simulink model "vtol50kg_airframe"  (R2024b)
settings: Solver=FixedStepAuto  StartTime=0  StopTime=200  FixedStep=5/1000  RelTol=1e-3
model workspace (MAT data in the model file):
  Sig = Simulink.Signal
  Sig.Dimensions = -1
  Sig.DimensionsMode = 'auto'
  Sig.Complexity = 'auto'
  Sig.SampleTime = -1
  Sig.SamplingMode = 'auto'
  Sig.DataType = 'auto'
  Sig1 = Simulink.Signal
  Sig1.Dimensions = -1
  Sig1.DimensionsMode = 'auto'
  Sig1.Complexity = 'auto'
  Sig1.SampleTime = -1
  Sig1.SamplingMode = 'auto'
  Sig1.DataType = 'auto'
  Sig2 = Simulink.Signal
  Sig2.Dimensions = -1
  Sig2.DimensionsMode = 'auto'
  Sig2.Complexity = 'auto'
  Sig2.SampleTime = -1
  Sig2.SamplingMode = 'auto'
  Sig2.DataType = 'auto'
  Sig3 = Simulink.Signal
  Sig3.Dimensions = -1
  Sig3.DimensionsMode = 'auto'
  Sig3.Complexity = 'auto'
  Sig3.SampleTime = -1
  Sig3.SamplingMode = 'auto'
  Sig3.DataType = 'auto'
  Sig4 = Simulink.Signal
  Sig4.Dimensions = -1
  Sig4.DimensionsMode = 'auto'
  Sig4.Complexity = 'auto'
  Sig4.SampleTime = -1
  Sig4.SamplingMode = 'auto'
  Sig4.DataType = 'auto'
  Sig5 = Simulink.Signal
  Sig5.Dimensions = -1
  Sig5.DimensionsMode = 'auto'
  Sig5.Complexity = 'auto'
  Sig5.SampleTime = -1
  Sig5.SamplingMode = 'auto'
  Sig5.DataType = 'auto'
  Sig6 = Simulink.Signal
  Sig6.Dimensions = -1
  Sig6.DimensionsMode = 'auto'
  Sig6.Complexity = 'auto'
  Sig6.SampleTime = -1
  Sig6.SamplingMode = 'auto'
  Sig6.DataType = 'auto'
values from neighbouring files (symbols this model uses):
  aerody =     [vtol50kg_airframe_data.mat]    (also in vtol50kg_airframe_init.m = init_aerody; vtol50kg_initdata.m = init_aerody)
  engine =     [vtol50kg_airframe_data.mat]    (also in vtol50kg_airframe_init.m = init_engine; vtol50kg_initdata.m = init_engine)
  mass =     [vtol50kg_airframe_data.mat]    (also in vtol50kg_airframe_init.m = init_weight; vtol50kg_initdata.m = init_weight)
  motor =     [vtol50kg_airframe_data.mat]    (also in vtol50kg_airframe_init.m = init_motor; vtol50kg_initdata.m = init_motor)
  payload =     [vtol50kg_airframe_data.mat]    (also in vtol50kg_airframe_init.m = init_payload; vtol50kg_initdata.m = init_payload)
undefined symbols (not defined in the file or in its folder): convertTo, datetime, Earth, F, Light, MIL, plant, WGS84, WMM2020
libraries: aerolibconvert2 x5, aerolibasang x5, aerolibwind2 x3, aerolibactuator x2, shared6dof x1, matrix_library x1, aerolibatmos2 x1, aerolibtransform2 x1, aerolibgravity2 x1
(part 1 of 2)
settings Model: DataDictionary=nextpilot_datadict.sldd  PauseTimes=10  Creator=zhanfuyu  LastModifiedBy=CETCA
settings OptimizationCC: BlockReduction=off  OptimizeBlockIOStorage=off  BufferReuse=off  ReuseModelBlockBuffer=off
settings DebuggingCC: AlgebraicLoopMsg=none
settings RTWCC: GPUComputeCapability=3.5

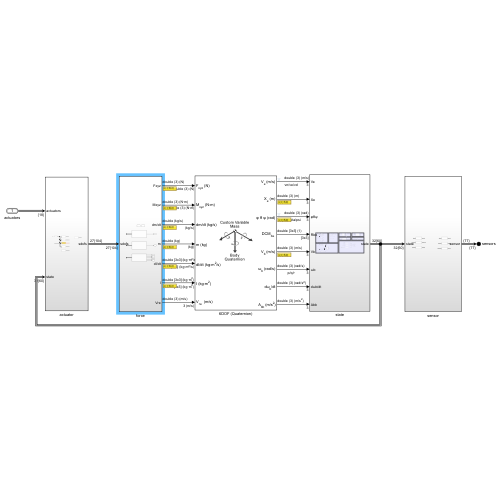
[thumbnail: Simulink's stored preview of the top-level diagram]
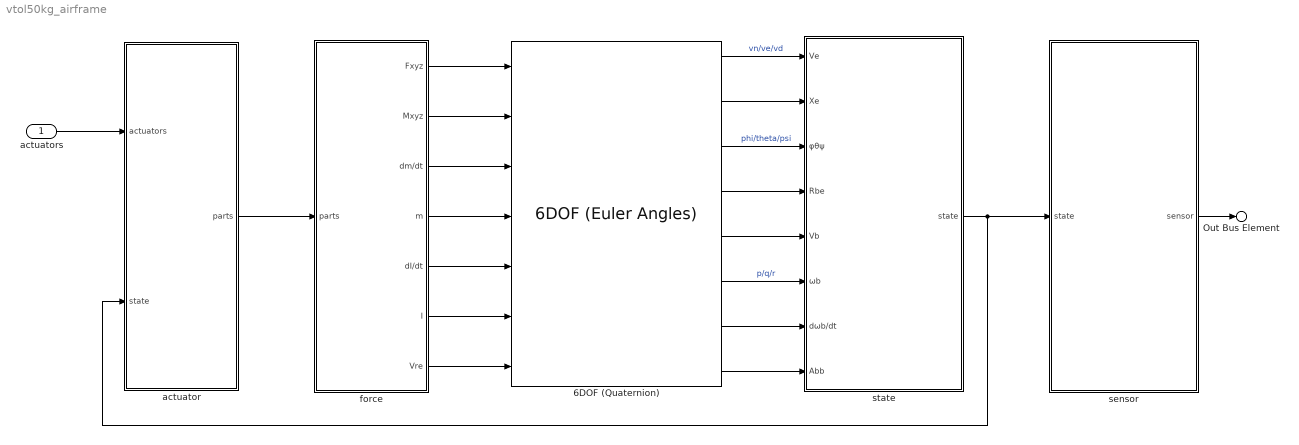
== system vtol50kg_airframe ==
  actuators : Inport  OutDataTypeStr=Bus: actuator_outputs_s
  6DOF (Quaternion) : shared6dof/6DOF (Euler Angles)  units=Metric (MKS)  mtype=Custom Variable  rep=Quaternion  xme_0=[0 0 0]  Vm_0=plant.init.vx_vy_vz  eul_0=plant.init.phi_theta_psi  pm_0=plant.init.p_q_r  mass_0=47  mass_e=0.5  mass_f=2.0  inertia=mass.emtpy_inertia  inertia_e=eye(3)  inertia_f=2*eye(3)  k_quat=1.0  vre_flag=on  abi_flag=off  aMode=0  xme_statename=''  Vm_statename=''  eul_statename=''  quat_statename=''  pm_statename=''  mass_statename=''
      settings: LibrarySourceBlock=aerolib6dof2/6DOF (Quaternion)
  actuator : Subsystem
  force : Subsystem
  sensor : Subsystem
  state : Subsystem
  Out Bus Element : Outport  PortName=sensors
  wires:
  state/1(state) -> actuator/2(state), sensor/1(state)
  sensor/1(sensor) -> Out Bus Element/1
  actuators/1 -> actuator/1(actuators)
  actuator/1(parts) -> force/1(parts)
  6DOF (Quaternion)/1 -> state/1(Ve)  "vn/ve/vd"
  6DOF (Quaternion)/2 -> state/2(Xe)
  6DOF (Quaternion)/3 -> state/3(φθψ)  "phi/theta/psi"
  6DOF (Quaternion)/4 -> state/4(Rbe)
  6DOF (Quaternion)/5 -> state/5(Vb)
  6DOF (Quaternion)/6 -> state/6(ωb)  "p/q/r"
  6DOF (Quaternion)/7 -> state/7(dωb/dt)
  6DOF (Quaternion)/8 -> state/8(Abb)
  force/1(Fxyz) -> 6DOF (Quaternion)/1
  force/2(Mxyz) -> 6DOF (Quaternion)/2
  force/3(dm/dt) -> 6DOF (Quaternion)/3
  force/4(m) -> 6DOF (Quaternion)/4
  force/5(dI/dt) -> 6DOF (Quaternion)/5
  force/6(I) -> 6DOF (Quaternion)/6
  force/7(Vre) -> 6DOF (Quaternion)/7

== system vtol50kg_airframe/actuator ==
  Bus Element In1 : Inport  PortName=actuators  Element=output
  Bus Element In : Inport  Port=2  PortName=state
  Subsystem : Subsystem
  battery : Subsystem
  engine : Subsystem
  fixed wing : Subsystem
  landgear : Subsystem
  payload : Subsystem
  rotor copter : Subsystem
  Bus Element Out : Outport  PortName=parts  Element=aerody
  Bus Element Out1 : Outport  PortName=parts  Element=rotor
  Bus Element Out2 : Outport  PortName=parts  Element=engine
  Bus Element Out3 : Outport  PortName=parts  Element=landgear
  Bus Element Out4 : Outport  PortName=parts  Element=battery
  Bus Element Out5 : Outport  PortName=parts  Element=payload
  wires:
  Bus Element In1/1 -> Subsystem/1(actuator)
  Subsystem/1(command) -> landgear/1(cmd), engine/1(cmd), rotor copter/1(cmd), fixed wing/1(cmd)
  Bus Element In/1 -> landgear/2(state), fixed wing/2(state), rotor copter/2(state), engine/2(state)
  fixed wing/1(aerody) -> Bus Element Out/1
  rotor copter/1(rotor) -> Bus Element Out1/1
  engine/1(engine) -> Bus Element Out2/1
  landgear/1(landgear) -> Bus Element Out3/1
  battery/1(battery) -> Bus Element Out4/1
  payload/1(payload) -> Bus Element Out5/1

== system vtol50kg_airframe/force ==
  BusElementIn : Inport  PortName=parts
  BusElementIn1 : Inport  PortName=parts
  BusElementIn2 : Inport  PortName=parts
  Force : Subsystem
  Goto Tag Visibility : GotoTagVisibility  GotoTag=mass
  Goto Tag Visibility1 : GotoTagVisibility  GotoTag=cog
  "Mass " : Subsystem
  Moment : Subsystem
  Fxyz : Outport
  Mxyz : Outport  Port=2
  dm/dt : Outport  Port=3
  m : Outport  Port=4
  dI/dt : Outport  Port=5
  I : Outport  Port=6
  Vre : Outport  Port=7
  wires:
  Force/1(Fxyz) -> Fxyz/1  "Fxzy"
  Moment/1(Mxyz) -> Mxyz/1  "Mxyz"
  BusElementIn/1 -> Force/1(parts)
  BusElementIn1/1 -> Moment/1(parts)
  BusElementIn2/1 -> "Mass "/1(parts)
  "Mass "/1(dM/dt) -> dm/dt/1
  "Mass "/2(M) -> m/1
  "Mass "/3(dI/dt) -> dI/dt/1
  "Mass "/4(I) -> I/1
  "Mass "/5(Vre) -> Vre/1

== system vtol50kg_airframe/sensor ==
  Bus Element In{,1..5} (6 alike) : Inport  PortName=state
  accel : Subsystem
  airspeed : Subsystem
  baro : Subsystem
  gps : Subsystem
  gyro : Subsystem
  mag : Subsystem
  Bus Element Out1 : Outport  PortName=sensor  Element=gps
  Bus Element Out3 : Outport  PortName=sensor  Element=gyro
  Bus Element Out4 : Outport  PortName=sensor  Element=accel
  Bus Element Out : Outport  PortName=sensor  Element=mag
  Bus Element Out2 : Outport  PortName=sensor  Element=baro
  Bus Element Out5 : Outport  PortName=sensor  Element=dpressure
  wires:
  Bus Element In/1 -> gps/1(state)
  Bus Element In1/1 -> mag/1(state)
  mag/1(mag) -> Bus Element Out/1
  gps/1(gps) -> Bus Element Out1/1
  baro/1(baro) -> Bus Element Out2/1
  Bus Element In2/1 -> baro/1(state)
  Bus Element In3/1 -> gyro/1(state)
  gyro/1(gyro) -> Bus Element Out3/1
  Bus Element In4/1 -> accel/1(state)
  accel/1(accel) -> Bus Element Out4/1
  Bus Element In5/1 -> airspeed/1(state)
  airspeed/1(dpressure) -> Bus Element Out5/1

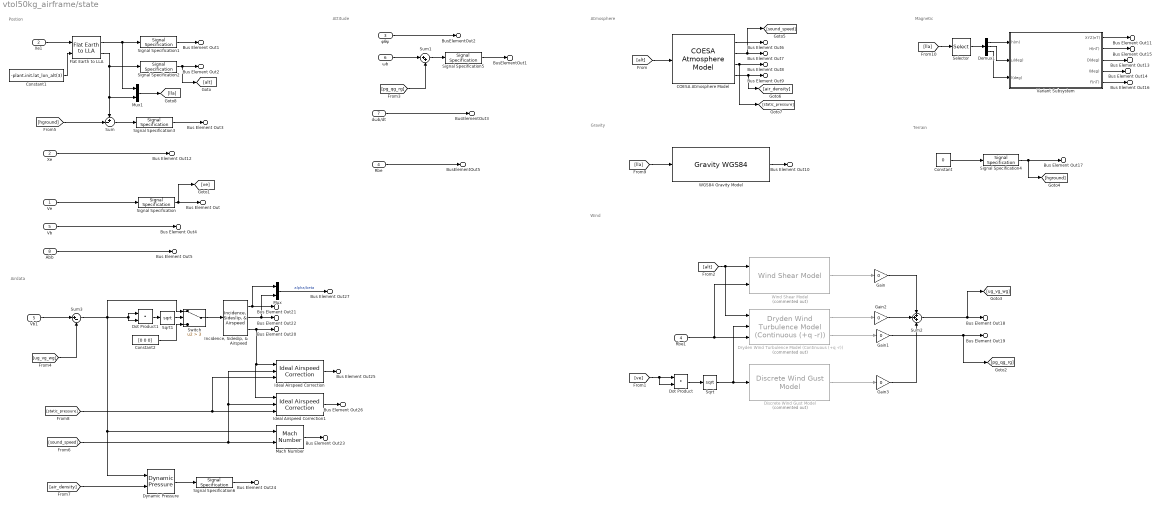
== system vtol50kg_airframe/state ==
  note: Postion
  note: Attitude
  note: Atmosphere
  note: Gravity
  note: Magnetic
  note: Terrain
  note: Wind
  note: Airdata
  Ve : Inport
  Xe : Inport  Port=2
  φθψ : Inport  Port=3
  Rbe : Inport  Port=4
  Vb : Inport  Port=5
  ωb : Inport  Port=6
  dωb/dt : Inport  Port=7
  Abb : Inport  Port=8
  COESA Atmosphere Model : aerolibatmos2/COESA Atmosphere Model  units=Metric (MKS)  spec=1976 COESA-extended U.S. Standard Atmosphere  model=Profile  profile_var=High temperature  profile_percent=1%  profile_alt=5 km (16404 ft)  envelope_var=High temperature  envelope_percent=1%  action=Warning
  Constant : Constant  Value=0
  Constant1 : Constant  Value=-plant.init.lat_lon_alt(3)
  Constant2 : Constant  Value=[0 0 0]
  Demux1 : Demux  Outputs=3
  Discrete Wind Gust Model : aerolibwind2/Discrete Wind Gust Model  Commented=on  units=Metric (MKS)  Gx=on  Gy=on  Gz=on  t_0=5  d_m=[120 120 80]  v_m=[3.5 3.5 3.0]
  Dot Product : DotProduct  OutDataTypeStr=Inherit: Inherit via internal rule
  Dot Product1 : DotProduct  OutDataTypeStr=Inherit: Inherit via internal rule
  Dryden Wind Turbulence Model (Continuous (+q -r)) : aerolibwind2/Dryden Wind Turbulence Model  (Continuous (+q -r))  Commented=on  units=Metric (MKS)  spec=MIL-F-8785C  model=Continuous Dryden (+q -r)  W20=15  Wdeg=0  TurbProb=10^-2 - Light  L_high=533.4  Wingspan=10  ts=0.1  Seed=[23341 23342 23343 23344]  T_on=on
  Dynamic Pressure : aerolibasang/Dynamic Pressure
  Flat Earth to LLA : aerolibtransform2/Flat Earth to LLA  units=Metric (MKS)  ptype=Earth (WGS84)  F=1/298.257223563  R=6378137  refPosPort=off  LL0=plant.init.lat_lon_alt(1:2)  psi=0
  Gain{,1..3} (4 alike) : Gain  Gain=0
  Ideal Airspeed Correction : aerolibasang/Ideal Airspeed Correction  units=Metric (MKS)  vel_in=TAS  vel_out_tas=CAS  vel_out_eas=TAS  vel_out_cas=TAS  method=Table Lookup  SubOnly=off  action=None
  Ideal Airspeed Correction1 : aerolibasang/Ideal Airspeed Correction  units=Metric (MKS)  vel_in=TAS  vel_out_tas=EAS  vel_out_eas=TAS  vel_out_cas=TAS  method=Table Lookup  SubOnly=off  action=None
  "Incidence, Sideslip, & Airspeed" : aerolibasang/Incidence, Sideslip, & Airspeed
  Mach Number : aerolibasang/Mach Number
  Mux : Mux  Inputs=2
  Mux1 : Mux  Inputs=2
  Rbe1 : InportShadow  Port=4
  Selector : Selector  InputPortWidth=3  IndexOptions=Index vector (dialog)  Indices=[3 1 2]  OutputSizes=1
  Signal Specification : SignalSpecification  Unit=m/s
  Signal Specification1 : SignalSpecification  Unit=deg
  Signal Specification2 : SignalSpecification  Unit=m
  Signal Specification3 : SignalSpecification  Unit=m
  Signal Specification4 : SignalSpecification  Unit=m
  Signal Specification5 : SignalSpecification  Unit=rad/s
  Signal Specification6 : SignalSpecification  Unit=Pa
  Sqrt : Sqrt
  Sqrt1 : Sqrt
  Sum : Sum  Inputs=+-|
  Sum1 : Sum  Inputs=|++
  Sum2 : Sum  Inputs=+++
  Sum3 : Sum  Inputs=|+-
  Switch : Switch  Criteria=u2 > Threshold  Threshold=3  SaturateOnIntegerOverflow=off  InputSameDT=off
  Variant Subsystem : Subsystem  Variant=on
  Vb1 : InportShadow  Port=5
  "WGS84 Gravity Model  " : GravityWGS84
  Wind Shear Model : aerolibwind2/Wind Shear Model  Commented=on  units=Metric (MKS)  phase=Category C - Terminal Flight Phase  W_20=15  Wdeg=0
  Xe1 : InportShadow  Port=2
  Bus Element Out1 : Outport  PortName=state  Element=aircraft.position.lat_lon
  Bus Element Out2 : Outport  PortName=state  Element=aircraft.position.alt
  Bus Element Out3 : Outport  PortName=state  Element=aircraft.position.agl
  Bus Element Out12 : Outport  PortName=state  Element=aircraft.position.pn_pe_pd
  Bus Element Out : Outport  PortName=state  Element=aircraft.position.vn_ve_vd
  Bus Element Out4 : Outport  PortName=state  Element=aircraft.position.ub_vb_wb
  Bus Element Out5 : Outport  PortName=state  Element=aircraft.position.ax_ay_az
  BusElementOut2 : Outport  PortName=state  Element=aircraft.attitude.phi_theta_psi
  BusElementOut1 : Outport  PortName=state  Element=aircraft.attitude.p_q_r
  BusElementOut3 : Outport  PortName=state  Element=aircraft.attitude.pdot_qdot_rdot
  BusElementOut5 : Outport  PortName=state  Element=aircraft.attitude.Rbe
  Bus Element Out20 : Outport  PortName=state  Element=aircraft.airdata.airspeed
  Bus Element Out21 : Outport  PortName=state  Element=aircraft.airdata.alpha
  Bus Element Out22 : Outport  PortName=state  Element=aircraft.airdata.beta
  Bus Element Out23 : Outport  PortName=state  Element=aircraft.airdata.mach
  Bus Element Out24 : Outport  PortName=state  Element=aircraft.airdata.qbar
  Bus Element Out25 : Outport  PortName=state  Element=aircraft.airdata.airspeed_cali
  Bus Element Out26 : Outport  PortName=state  Element=aircraft.airdata.airspeed_equ
  Bus Element Out27 : Outport  PortName=state  Element=aircraft.airdata.alpha_beta
  Bus Element Out6 : Outport  PortName=state  Element=environ.atmosphere.temperature
  Bus Element Out7 : Outport  PortName=state  Element=environ.atmosphere.soundspeed
  Bus Element Out8 : Outport  PortName=state  Element=environ.atmosphere.pressure
  Bus Element Out9 : Outport  PortName=state  Element=environ.atmosphere.density
  Bus Element Out10 : Outport  PortName=state  Element=environ.gravity.xyz
  Bus Element Out11 : Outport  PortName=state  Element=environ.magnetic.xyz
  Bus Element Out13 : Outport  PortName=state  Element=environ.magnetic.declination
  Bus Element Out14 : Outport  PortName=state  Element=environ.magnetic.inclination
  Bus Element Out15 : Outport  PortName=state  Element=environ.magnetic.hor_intensity
  Bus Element Out16 : Outport  PortName=state  Element=environ.magnetic.total_intensity
  Bus Element Out17 : Outport  PortName=state  Element=environ.terrain.hground
  Bus Element Out18 : Outport  PortName=state  Element=environ.wind.ug_vg_wg
  Bus Element Out19 : Outport  PortName=state  Element=environ.wind.pg_qg_rg
  wires:
  Signal Specification6/1 -> Bus Element Out24/1
  Signal Specification5/1 -> BusElementOut1/1
  Gain3/1 -> Sum2/3
  Gain2/1 -> Sum2/2
  Gain/1 -> Sum2/1
  Mux/1 -> Bus Element Out27/1  "alpha/beta"
  Ideal Airspeed Correction1/1 -> Bus Element Out26/1
  Ideal Airspeed Correction/1 -> Bus Element Out25/1
  [static_pressure] -> Ideal Airspeed Correction1/3, Ideal Airspeed Correction/3
  [air_density] -> Dynamic Pressure/2
  Dynamic Pressure/1 -> Signal Specification6/1
  Mach Number/1 -> Bus Element Out23/1
  [sound_speed] -> Mach Number/2, Ideal Airspeed Correction/2, Ideal Airspeed Correction1/2
  "Incidence, Sideslip, & Airspeed"/1 -> Bus Element Out21/1, Mux/1
  "Incidence, Sideslip, & Airspeed"/2 -> Bus Element Out22/1, Mux/2
  "Incidence, Sideslip, & Airspeed"/3 -> Bus Element Out20/1, Ideal Airspeed Correction1/1, Ideal Airspeed Correction/1
  Sum3/1 -> Dot Product1/1, Dot Product1/2, Switch/1, Mach Number/1, Dynamic Pressure/1
  [ug_vg_wg] -> Sum3/2
  Vb1/1 -> Sum3/1
  Gain1/1 -> Bus Element Out19/1, [pg_qg_rg]
  Wind Shear Model/1 -> Gain/1
  Sum2/1 -> Bus Element Out18/1, [ug_vg_wg]
  Sqrt/1 -> Discrete Wind Gust Model/1, Dryden Wind Turbulence Model (Continuous (+q -r))/2
  Dot Product/1 -> Sqrt/1
  [ve] -> Dot Product/1, Dot Product/2
  [alt] -> Dryden Wind Turbulence Model (Continuous (+q -r))/1, Wind Shear Model/1
  Rbe1/1 -> Dryden Wind Turbulence Model (Continuous (+q -r))/3, Wind Shear Model/2
  Dryden Wind Turbulence Model (Continuous (+q -r))/2 -> Gain1/1
  Discrete Wind Gust Model/1 -> Gain3/1
  Dryden Wind Turbulence Model (Continuous (+q -r))/1 -> Gain2/1
  Signal Specification4/1 -> Bus Element Out17/1, [hground]
  Constant/1 -> Signal Specification4/1
  Variant Subsystem/5(F(nT)) -> Bus Element Out16/1
  Variant Subsystem/2(H(nT)) -> Bus Element Out15/1
  Variant Subsystem/4(I(deg)) -> Bus Element Out14/1
  Variant Subsystem/3(D(deg)) -> Bus Element Out13/1
  Demux1/3 -> Variant Subsystem/3(l(deg))
  Demux1/2 -> Variant Subsystem/2(μ(deg))
  Demux1/1 -> Variant Subsystem/1(h(m))
  Selector/1 -> Demux1/1
  [lla] -> Selector/1
  "WGS84 Gravity Model  "/1 -> Bus Element Out10/1
  [lla] -> "WGS84 Gravity Model  "/1
  COESA Atmosphere Model/4 -> Bus Element Out9/1, [air_density]
  COESA Atmosphere Model/3 -> Bus Element Out8/1, [static_pressure]
  COESA Atmosphere Model/2 -> Bus Element Out7/1, [sound_speed]
  COESA Atmosphere Model/1 -> Bus Element Out6/1
  [alt] -> COESA Atmosphere Model/1
  Xe/1 -> Bus Element Out12/1
  dωb/dt/1 -> BusElementOut3/1
  [pg_qg_rg] -> Sum1/2
  Sum1/1 -> Signal Specification5/1
  ωb/1 -> Sum1/1
  Rbe/1 -> BusElementOut5/1
  φθψ/1 -> BusElementOut2/1
  Abb/1 -> Bus Element Out5/1
  Vb/1 -> Bus Element Out4/1
  [hground] -> Sum/2
  Signal Specification3/1 -> Bus Element Out3/1
  Sum/1 -> Signal Specification3/1
  Signal Specification2/1 -> Bus Element Out2/1, [alt]
  Signal Specification1/1 -> Bus Element Out1/1
  Signal Specification/1 -> Bus Element Out/1, [ve]
  Ve/1 -> Signal Specification/1
  Xe1/1 -> Flat Earth to LLA/1
  Flat Earth to LLA/1 -> Mux1/1, Signal Specification1/1
  Flat Earth to LLA/2 -> Sum/1, Mux1/2, Signal Specification2/1
  Constant1/1 -> Flat Earth to LLA/2
  Mux1/1 -> [lla]
  Variant Subsystem/1(XYZ(nT)) -> Bus Element Out11/1
  Switch/1 -> "Incidence, Sideslip, & Airspeed"/1
  Constant2/1 -> Switch/3
  Sqrt1/1 -> Switch/2
  Dot Product1/1 -> Sqrt1/1

== system vtol50kg_airframe/actuator/Subsystem ==
  actuator : Inport
  Demux : Demux  Outputs=16
  Bus Element Out1 : Outport  PortName=command  Element=pwm_mc_rf
  Bus Element Out2 : Outport  PortName=command  Element=pwm_mc_lb
  Bus Element Out3 : Outport  PortName=command  Element=pwm_mc_lf
  Bus Element Out4 : Outport  PortName=command  Element=pwm_mc_rb
  Bus Element Out5 : Outport  PortName=command  Element=pwm05
  Bus Element Out6 : Outport  PortName=command  Element=pwm06
  Bus Element Out7 : Outport  PortName=command  Element=pwm07
  Bus Element Out8 : Outport  PortName=command  Element=pwm08
  Bus Element Out9 : Outport  PortName=command  Element=pwm_fw_la
  Bus Element Out10 : Outport  PortName=command  Element=pwm_fw_ra
  Bus Element Out11 : Outport  PortName=command  Element=pwm_fw_le
  Bus Element Out12 : Outport  PortName=command  Element=pwm_fw_re
  Bus Element Out13 : Outport  PortName=command  Element=pwm_fw_lr
  Bus Element Out14 : Outport  PortName=command  Element=pwm_fw_rr
  Bus Element Out15 : Outport  PortName=command  Element=pwm_fw_throttle
  Bus Element Out16 : Outport  PortName=command  Element=pwm16
  wires:
  actuator/1 -> Demux/1
  Demux/1 -> Bus Element Out1/1
  Demux/2 -> Bus Element Out2/1
  Demux/3 -> Bus Element Out3/1
  Demux/4 -> Bus Element Out4/1
  Demux/5 -> Bus Element Out5/1
  Demux/6 -> Bus Element Out6/1
  Demux/7 -> Bus Element Out7/1
  Demux/8 -> Bus Element Out8/1
  Demux/9 -> Bus Element Out9/1
  Demux/10 -> Bus Element Out10/1
  Demux/11 -> Bus Element Out11/1
  Demux/12 -> Bus Element Out12/1
  Demux/13 -> Bus Element Out13/1
  Demux/14 -> Bus Element Out14/1
  Demux/15 -> Bus Element Out15/1
  Demux/16 -> Bus Element Out16/1

== system vtol50kg_airframe/actuator/battery ==
  Constant : Constant
  Constant1 : Constant  Value=50
  Bus Element Out : Outport  PortName=battery  Element=voltage
  Bus Element Out1 : Outport  PortName=battery  Element=soc
  wires:
  Constant/1 -> Bus Element Out1/1
  Constant1/1 -> Bus Element Out/1

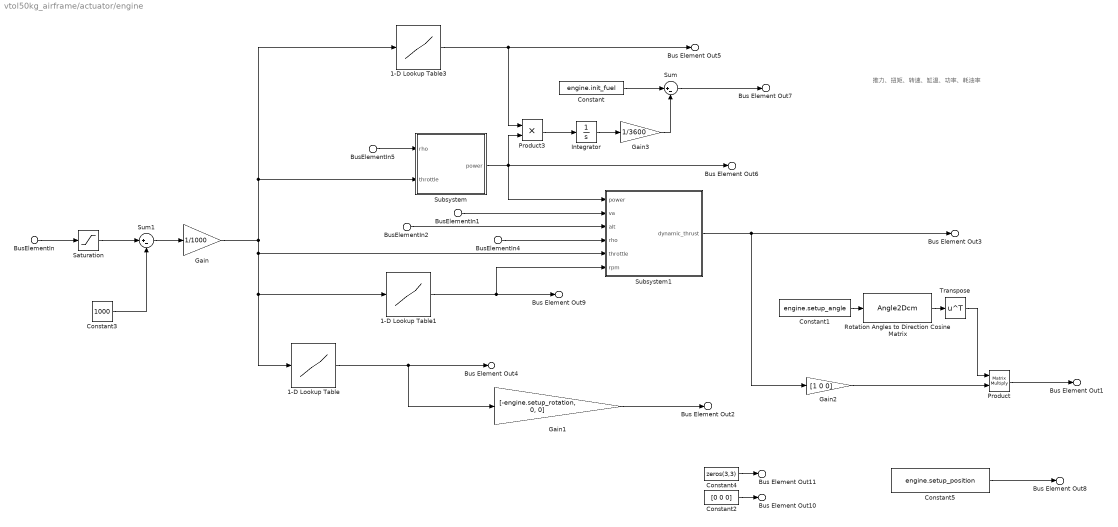
== system vtol50kg_airframe/actuator/engine ==
  note: 推力、扭矩、转速、缸温、功率、耗油率
  BusElementIn : Inport  PortName=cmd  Element=pwm_fw_throttle
  BusElementIn1 : Inport  Port=2  PortName=state  Element=aircraft.airdata.airspeed
  BusElementIn2 : Inport  Port=2  PortName=state  Element=aircraft.position.alt
  BusElementIn4 : Inport  Port=2  PortName=state  Element=environ.atmosphere.density
  BusElementIn5 : Inport  Port=2  PortName=state  Element=environ.atmosphere.density
  1-D Lookup Table : Lookup_n-D  NumberOfTableDimensions=1  BreakpointsForDimension1=engine.torque.delta  IndexSearchMethod=Linear search  BeginIndexSearchUsingPreviousIndexResult=on  Table=engine.torque.moment  ExtrapMethod=Clip  InternalRulePriority=Speed  RndMeth=Simplest
  1-D Lookup Table1 : Lookup_n-D  NumberOfTableDimensions=1  BreakpointsForDimension1=engine.torque.delta  IndexSearchMethod=Linear search  BeginIndexSearchUsingPreviousIndexResult=on  Table=engine.torque.rpm  ExtrapMethod=Clip  InternalRulePriority=Speed  RndMeth=Simplest
  1-D Lookup Table3 : Lookup_n-D  NumberOfTableDimensions=1  BreakpointsForDimension1=engine.torque.delta  IndexSearchMethod=Linear search  BeginIndexSearchUsingPreviousIndexResult=on  Table=engine.torque.fuel_cons_rate  ExtrapMethod=Clip  InternalRulePriority=Speed  RndMeth=Simplest
  Constant : Constant  Value=engine.init_fuel
  Constant1 : Constant  Value=engine.setup_angle
  Constant2 : Constant  Value=[0 0 0]
  Constant3 : Constant  Value=1000
  Constant4 : Constant  Value=zeros(3,3)
  Constant5 : Constant  Value=engine.setup_position
  Gain : Gain  Gain=1/1000
  Gain1 : Gain  Gain=[-engine.setup_rotation, 0, 0]
  Gain2 : Gain  Gain=[1 0 0]
  Gain3 : Gain  Gain=1/3600
  Integrator : Integrator
  Product : Product  Multiplication=Matrix(*)
  Product3 : Product
  Rotation Angles to Direction Cosine Matrix : Angle2Dcm
      settings: AttributesFormatString=Rotation Order: %<rotationOrder>
  Saturation : Saturate  UpperLimit=2000  LowerLimit=1000
  Subsystem : Subsystem
  Subsystem1 : Subsystem
  Sum : Sum  Inputs=|+-
  Sum1 : Sum  Inputs=|+-
  Transpose : Math  Operator=transpose
  Bus Element Out3 : Outport  PortName=engine  Element=state.thrust
  Bus Element Out4 : Outport  PortName=engine  Element=state.toruqe
  Bus Element Out6 : Outport  PortName=engine  Element=state.power
  Bus Element Out9 : Outport  PortName=engine  Element=state.rpm
  Bus Element Out5 : Outport  PortName=engine  Element=state.fuel_com_rate
  Bus Element Out8 : Outport  PortName=engine  Element=Pxyz
  Bus Element Out1 : Outport  PortName=engine  Element=Fxyz
  Bus Element Out2 : Outport  PortName=engine  Element=Mxyz
  Bus Element Out7 : Outport  PortName=engine  Element=fuel_mass
  Bus Element Out10 : Outport  PortName=engine  Element=fuel_cog
  Bus Element Out11 : Outport  PortName=engine  Element=fuel_inertia
  wires:
  Constant/1 -> Sum/1
  Integrator/1 -> Gain3/1
  Rotation Angles to Direction Cosine Matrix/1 -> Transpose/1
  Constant1/1 -> Rotation Angles to Direction Cosine Matrix/1
  Gain1/1 -> Bus Element Out2/1
  1-D Lookup Table/1 -> Gain1/1, Bus Element Out4/1
  Constant3/1 -> Sum1/2
  Sum1/1 -> Gain/1
  Gain/1 -> Subsystem1/5(throttle), 1-D Lookup Table1/1, 1-D Lookup Table/1, 1-D Lookup Table3/1, Subsystem/2(throttle)
  1-D Lookup Table3/1 -> Bus Element Out5/1, Product3/1
  Product3/1 -> Integrator/1
  Sum/1 -> Bus Element Out7/1
  Constant5/1 -> Bus Element Out8/1
  BusElementIn5/1 -> Subsystem/1(rho)
  Subsystem/1(power) -> Subsystem1/1(power), Product3/2, Bus Element Out6/1
  BusElementIn4/1 -> Subsystem1/4(rho)
  BusElementIn1/1 -> Subsystem1/2(va)
  BusElementIn2/1 -> Subsystem1/3(alt)
  Subsystem1/1(dynamic_thrust) -> Bus Element Out3/1, Gain2/1
  Product/1 -> Bus Element Out1/1
  1-D Lookup Table1/1 -> Bus Element Out9/1, Subsystem1/6(rpm)
  Gain3/1 -> Sum/2
  BusElementIn/1 -> Saturation/1
  Constant2/1 -> Bus Element Out10/1
  Constant4/1 -> Bus Element Out11/1
  Transpose/1 -> Product/1
  Gain2/1 -> Product/2
  Saturation/1 -> Sum1/1

== system vtol50kg_airframe/actuator/fixed wing ==
  BusElementIn4 : Inport  PortName=cmd
  Bus Element In1 : Inport  Port=2  PortName=state
  actuator : Subsystem
  aerodynamics : Subsystem
  Bus Element Out1 : Outport  PortName=aerody
  wires:
  BusElementIn4/1 -> actuator/1(command)
  actuator/1(surface) -> aerodynamics/1(surface)
  Bus Element In1/1 -> aerodynamics/2(state)
  aerodynamics/1(aerody) -> Bus Element Out1/1

== system vtol50kg_airframe/actuator/landgear ==
  note: ASL：above sea level
      | AGL：above groud level
  BusElementIn : Inport  PortName=cmd
  BusElementIn1 : Inport  Port=2  PortName=state  Element=aircraft.position.agl
  BusElementIn3 : Inport  Port=2  PortName=state  Element=aircraft.position.vn_ve_vd
  Constant : Constant  Value=[0 0 0]
  Constant1 : Constant  Value=-0.5
  Constant2 : Constant  Value=0
  Gain : Gain  Gain=1e5
  Gain1 : Gain  Gain=[0,0,1]
  Gain2 : Gain  Gain=-1e4
  GreaterThan : RelationalOperator  Operator=<  OutDataTypeStr=boolean  RndMeth=Simplest  InputSameDT=off
  Selector : Selector  InputPortWidth=3  IndexOptions=Index vector (dialog)  Indices=3  OutputSizes=1
  Stop Simulation : Stop  Commented=on
  Sum : Sum  Inputs=|++
  Switch : Switch  Criteria=u2 > Threshold  SaturateOnIntegerOverflow=off  InputSameDT=off
  Switch1 : Switch  Criteria=u2 > Threshold  SaturateOnIntegerOverflow=off  InputSameDT=off
  Terminator : Terminator
  Bus Element Out3 : Outport  PortName=landgear  Element=Fxyz
  Bus Element Out1 : Outport  PortName=landgear  Element=Mxyz
  Bus Element Out2 : Outport  PortName=landgear  Element=Pxyz
  wires:
  Constant/1 -> Bus Element Out2/1, Bus Element Out1/1
  BusElementIn/1 -> Terminator/1
  BusElementIn1/1 -> Switch1/2, Switch1/3, Switch/2, GreaterThan/1
  Constant1/1 -> GreaterThan/2
  GreaterThan/1 -> Stop Simulation/1
  Gain1/1 -> Bus Element Out3/1
  Gain/1 -> Sum/1
  Sum/1 -> Gain1/1
  BusElementIn3/1 -> Selector/1
  Gain2/1 -> Sum/2
  Switch/1 -> Gain2/1
  Constant2/1 -> Switch/1, Switch1/1
  Selector/1 -> Switch/3
  Switch1/1 -> Gain/1

== system vtol50kg_airframe/actuator/payload ==
  Constant : Constant  Value=payload.inertia
  Constant1 : Constant  Value=payload.cog
  Constant2 : Constant  Value=payload.weight
  Bus Element Out : Outport  PortName=payload  Element=mcog
  Bus Element Out1 : Outport  PortName=payload  Element=inertia
  Bus Element Out2 : Outport  PortName=payload  Element=mass
  wires:
  Constant1/1 -> Bus Element Out/1
  Constant/1 -> Bus Element Out1/1
  Constant2/1 -> Bus Element Out2/1

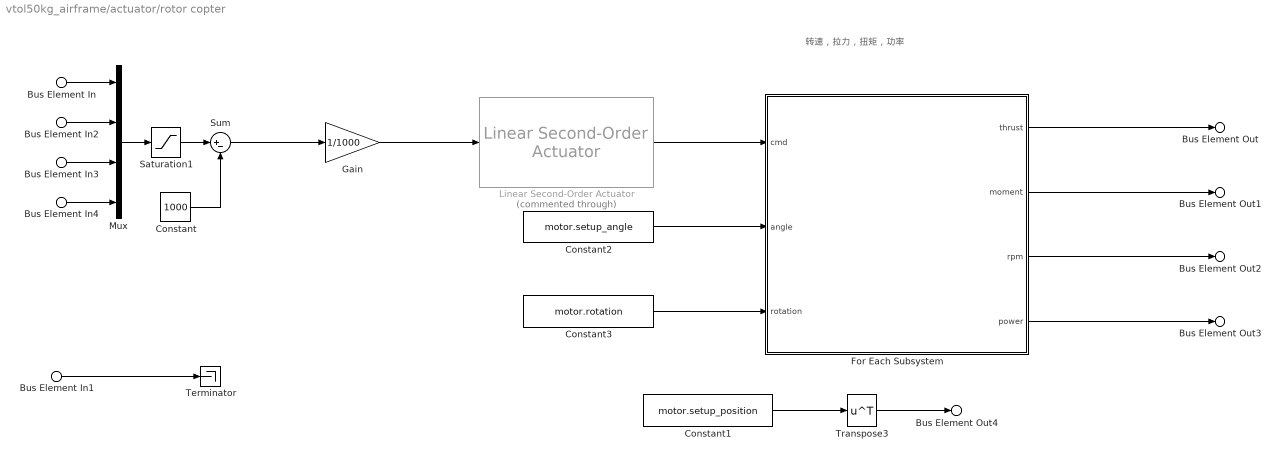
== system vtol50kg_airframe/actuator/rotor copter ==
  note: 转速，拉力，扭矩，功率
  Bus Element In : Inport  PortName=cmd  Element=pwm_mc_rf
  Bus Element In2 : Inport  PortName=cmd  Element=pwm_mc_lb
  Bus Element In3 : Inport  PortName=cmd  Element=pwm_mc_lf
  Bus Element In4 : Inport  PortName=cmd  Element=pwm_mc_rb
  Bus Element In1 : Inport  Port=2  PortName=state
  Constant : Constant  Value=1000
  Constant1 : Constant  Value=motor.setup_position
  Constant2 : Constant  Value=motor.setup_angle
  Constant3 : Constant  Value=motor.rotation
  For Each Subsystem : Subsystem  TreatAsAtomicUnit=on
  Gain : Gain  Gain=1/1000
  Linear Second-Order Actuator : aerolibactuator/Linear Second-Order Actuator  Commented=through  wn_fin=1  z_fin=0.3  fin_act_0=0  fin_act_vel=0
  Mux : Mux
  Saturation1 : Saturate  UpperLimit=2000  LowerLimit=1000
  Sum : Sum  Inputs=|+-
  Terminator : Terminator
  Transpose3 : Math  Operator=transpose
  Bus Element Out2 : Outport  PortName=rotor  Element=state.rpm
  Bus Element Out3 : Outport  PortName=rotor  Element=state.power
  Bus Element Out : Outport  PortName=rotor  Element=Fxyz
  Bus Element Out1 : Outport  PortName=rotor  Element=Mxyz
  Bus Element Out4 : Outport  PortName=rotor  Element=Pxyz
  wires:
  Bus Element In3/1 -> Mux/3
  Bus Element In2/1 -> Mux/2
  Bus Element In4/1 -> Mux/4
  Bus Element In/1 -> Mux/1
  Mux/1 -> Saturation1/1
  Constant/1 -> Sum/2
  Sum/1 -> Gain/1
  Gain/1 -> Linear Second-Order Actuator/1
  Constant2/1 -> For Each Subsystem/2(angle)
  Constant3/1 -> For Each Subsystem/3(rotation)
  For Each Subsystem/1(thrust) -> Bus Element Out/1
  For Each Subsystem/2(moment) -> Bus Element Out1/1
  For Each Subsystem/3(rpm) -> Bus Element Out2/1
  For Each Subsystem/4(power) -> Bus Element Out3/1
  Bus Element In1/1 -> Terminator/1
  Linear Second-Order Actuator/1 -> For Each Subsystem/1(cmd)
  Constant1/1 -> Transpose3/1
  Transpose3/1 -> Bus Element Out4/1
  Saturation1/1 -> Sum/1

== system vtol50kg_airframe/force/Force ==
  BusElementIn1 : Inport  PortName=parts  Element=aerody.Fxyz
  BusElementIn2 : Inport  PortName=parts  Element=rotor.Fxyz
  BusElementIn4 : Inport  PortName=parts  Element=engine.Fxyz
  BusElementIn3 : Inport  PortName=parts  Element=landgear.Fxyz
  Gain : Gain  Gain=[0 0 9.81]
  Reshape : Reshape
  Reshape1 : Reshape
  Sum : Sum  Inputs=5
  Sum3 : Sum  Inputs=1  CollapseMode=Specified dimension  CollapseDim=2
  Fxyz : Outport
  wires:
  BusElementIn2/1 -> Sum3/1
  BusElementIn4/1 -> Sum/3
  BusElementIn1/1 -> Sum/1
  Reshape/1 -> Fxyz/1
  Sum/1 -> Reshape/1
  [mass] -> Gain/1
  Sum3/1 -> Reshape1/1
  Reshape1/1 -> Sum/2
  Gain/1 -> Sum/5
  BusElementIn3/1 -> Sum/4

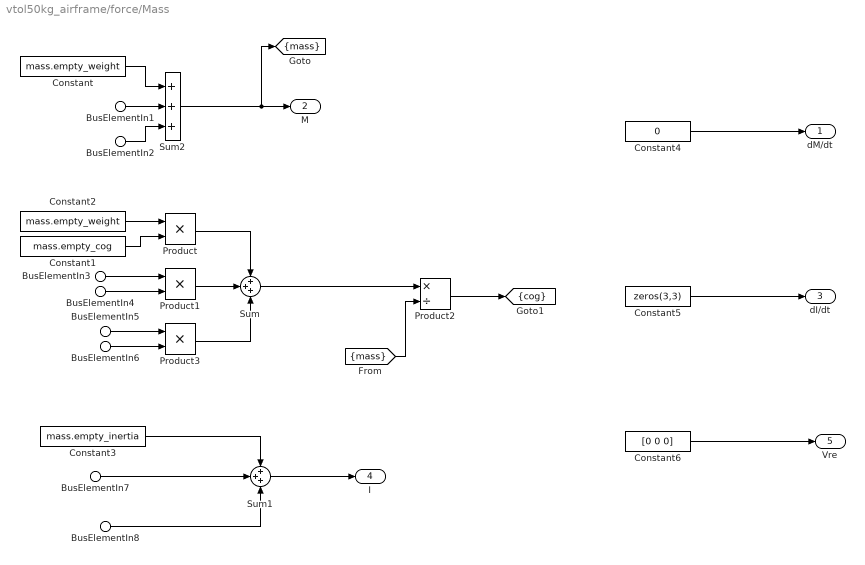
== system vtol50kg_airframe/force/Mass  ==
  BusElementIn2 : Inport  PortName=parts  Element=engine.fuel_mass
  BusElementIn5 : Inport  PortName=parts  Element=engine.fuel_mass
  BusElementIn6 : Inport  PortName=parts  Element=engine.fuel_cog
  BusElementIn8 : Inport  PortName=parts  Element=engine.fuel_inertia
  BusElementIn4 : Inport  PortName=parts  Element=payload.mcog
  BusElementIn7 : Inport  PortName=parts  Element=payload.inertia
  BusElementIn1 : Inport  PortName=parts  Element=payload.mass
  BusElementIn3 : Inport  PortName=parts  Element=payload.mass
  Constant : Constant  Value=mass.empty_weight
  Constant1 : Constant  Value=mass.empty_cog
  Constant2 : Constant  Value=mass.empty_weight
  Constant3 : Constant  Value=mass.empty_inertia
  Constant4 : Constant  Value=0
  Constant5 : Constant  Value=zeros(3,3)
  Constant6 : Constant  Value=[0 0 0]
  Product : Product
  Product1 : Product
  Product2 : Product  Inputs=*/
  Product3 : Product
  Sum : Sum  Inputs=3
  Sum1 : Sum  Inputs=3
  Sum2 : Sum  Inputs=3
  dM/dt : Outport
  M : Outport  Port=2
  dI/dt : Outport  Port=3
  I : Outport  Port=4
  Vre : Outport  Port=5
  tag scope: cog=scoped, mass=scoped
  wires:
  Constant/1 -> Sum2/1
  Sum2/1 -> M/1, [mass]
  BusElementIn1/1 -> Sum2/2
  BusElementIn2/1 -> Sum2/3
  Constant2/1 -> Product/1
  Product/1 -> Sum/1
  Product1/1 -> Sum/2
  BusElementIn3/1 -> Product1/1
  BusElementIn4/1 -> Product1/2
  Sum/1 -> Product2/1
  [mass] -> Product2/2
  Product2/1 -> [cog]
  Product3/1 -> Sum/3
  Constant1/1 -> Product/2
  BusElementIn5/1 -> Product3/1
  BusElementIn6/1 -> Product3/2
  Constant3/1 -> Sum1/1
  BusElementIn7/1 -> Sum1/2
  BusElementIn8/1 -> Sum1/3
  Sum1/1 -> I/1
  Constant6/1 -> Vre/1
  Constant4/1 -> dM/dt/1
  Constant5/1 -> dI/dt/1

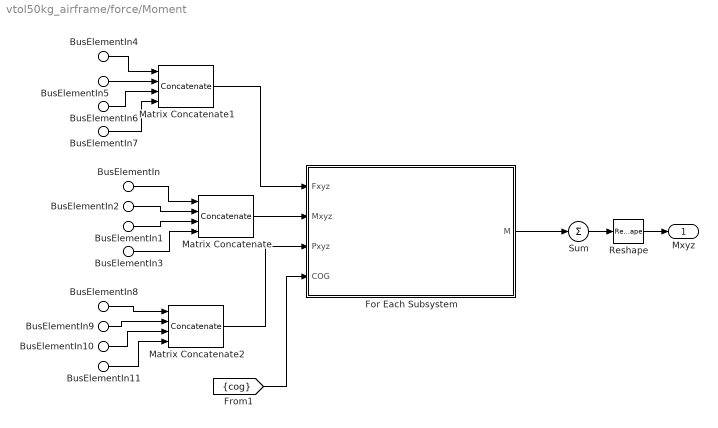
== system vtol50kg_airframe/force/Moment ==
  BusElementIn : Inport  PortName=parts  Element=aerody.Mxyz
  BusElementIn4 : Inport  PortName=parts  Element=aerody.Fxyz
  BusElementIn8 : Inport  PortName=parts  Element=aerody.Pxyz
  BusElementIn1 : Inport  PortName=parts  Element=engine.Mxyz
  BusElementIn6 : Inport  PortName=parts  Element=engine.Fxyz
  BusElementIn10 : Inport  PortName=parts  Element=engine.Pxyz
  BusElementIn2 : Inport  PortName=parts  Element=rotor.Mxyz
  BusElementIn5 : Inport  PortName=parts  Element=rotor.Fxyz
  BusElementIn9 : Inport  PortName=parts  Element=rotor.Pxyz
  BusElementIn3 : Inport  PortName=parts  Element=landgear.Mxyz
  BusElementIn7 : Inport  PortName=parts  Element=landgear.Fxyz
  BusElementIn11 : Inport  PortName=parts  Element=landgear.Pxyz
  For Each Subsystem : Subsystem  TreatAsAtomicUnit=on
  Matrix Concatenate : Concatenate  NumInputs=4  Mode=Multidimensional array  ConcatenateDimension=2
  Matrix Concatenate1 : Concatenate  NumInputs=4  Mode=Multidimensional array  ConcatenateDimension=2
  Matrix Concatenate2 : Concatenate  NumInputs=4  Mode=Multidimensional array  ConcatenateDimension=2
  Reshape : Reshape
  Sum : Sum  Inputs=1  CollapseMode=Specified dimension  CollapseDim=2
  Mxyz : Outport
  wires:
  For Each Subsystem/1(M) -> Sum/1
  Matrix Concatenate/1 -> For Each Subsystem/2(Mxyz)
  Matrix Concatenate1/1 -> For Each Subsystem/1(Fxyz)
  Matrix Concatenate2/1 -> For Each Subsystem/3(Pxyz)
  [cog] -> For Each Subsystem/4(COG)
  Sum/1 -> Reshape/1
  Reshape/1 -> Mxyz/1
  BusElementIn6/1 -> Matrix Concatenate1/3
  BusElementIn5/1 -> Matrix Concatenate1/2
  BusElementIn4/1 -> Matrix Concatenate1/1
  BusElementIn7/1 -> Matrix Concatenate1/4
  BusElementIn2/1 -> Matrix Concatenate/2
  BusElementIn1/1 -> Matrix Concatenate/3
  BusElementIn/1 -> Matrix Concatenate/1
  BusElementIn3/1 -> Matrix Concatenate/4
  BusElementIn9/1 -> Matrix Concatenate2/2
  BusElementIn8/1 -> Matrix Concatenate2/1
  BusElementIn10/1 -> Matrix Concatenate2/3
  BusElementIn11/1 -> Matrix Concatenate2/4

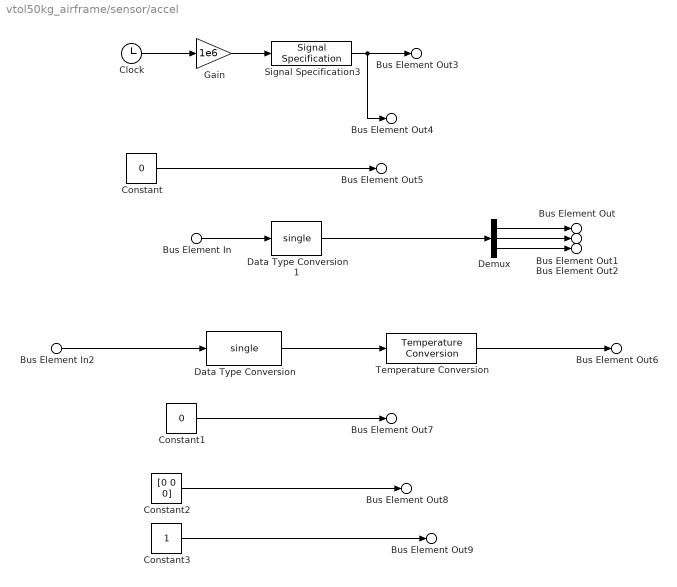
== system vtol50kg_airframe/sensor/accel ==
  Bus Element In2 : Inport  PortName=state  Element=environ.atmosphere.temperature
  Bus Element In : Inport  PortName=state  Element=aircraft.position.ax_ay_az
  Clock : Clock
  Constant : Constant  Value=0  OutDataTypeStr=uint32
  Constant1 : Constant  Value=0  OutDataTypeStr=uint32
  Constant2 : Constant  Value=[0 0 0]  OutDataTypeStr=uint8
  Constant3 : Constant  OutDataTypeStr=uint8
  Data Type Conversion : DataTypeConversion  OutDataTypeStr=single  SaturateOnIntegerOverflow=off  RndMeth=Floor
  Data Type Conversion1 : DataTypeConversion  OutDataTypeStr=single  SaturateOnIntegerOverflow=off  RndMeth=Floor
  Demux : Demux  Outputs=3
  Gain : Gain  Gain=1e6  OutDataTypeStr=uint64
  Signal Specification3 : SignalSpecification  Unit=µs
  Temperature Conversion : aerolibconvert2/Temperature Conversion  IU=K  OU=C
  Bus Element Out3 : Outport  PortName=accel  Element=timestamp
  Bus Element Out4 : Outport  PortName=accel  Element=timestamp_sample
  Bus Element Out5 : Outport  PortName=accel  Element=device_id
  Bus Element Out : Outport  PortName=accel  Element=x
  Bus Element Out1 : Outport  PortName=accel  Element=y
  Bus Element Out2 : Outport  PortName=accel  Element=z
  Bus Element Out6 : Outport  PortName=accel  Element=temperature
  Bus Element Out7 : Outport  PortName=accel  Element=error_count
  Bus Element Out8 : Outport  PortName=accel  Element=clip_counter
  Bus Element Out9 : Outport  PortName=accel  Element=samples
  wires:
  Constant3/1 -> Bus Element Out9/1
  Constant2/1 -> Bus Element Out8/1
  Bus Element In/1 -> Data Type Conversion1/1
  Demux/1 -> Bus Element Out/1
  Demux/2 -> Bus Element Out1/1
  Demux/3 -> Bus Element Out2/1
  Clock/1 -> Gain/1
  Signal Specification3/1 -> Bus Element Out4/1, Bus Element Out3/1
  Gain/1 -> Signal Specification3/1
  Constant/1 -> Bus Element Out5/1
  Constant1/1 -> Bus Element Out7/1
  Bus Element In2/1 -> Data Type Conversion/1
  Temperature Conversion/1 -> Bus Element Out6/1
  Data Type Conversion/1 -> Temperature Conversion/1
  Data Type Conversion1/1 -> Demux/1

== system vtol50kg_airframe/sensor/airspeed ==
  Bus Element In2 : Inport  PortName=state  Element=environ.atmosphere.temperature
  Bus Element In1 : Inport  PortName=state  Element=aircraft.airdata.qbar
  Clock : Clock
  Constant : Constant  Value=0  OutDataTypeStr=uint32
  Constant1 : Constant  Value=0  OutDataTypeStr=uint32
  Data Type Conversion : DataTypeConversion  OutDataTypeStr=single  SaturateOnIntegerOverflow=off  RndMeth=Floor
  Data Type Conversion1 : DataTypeConversion  OutDataTypeStr=single  SaturateOnIntegerOverflow=off  RndMeth=Floor
  Gain : Gain  Gain=1e6  OutDataTypeStr=uint64
  Signal Specification3 : SignalSpecification  Unit=µs
  Temperature Conversion : aerolibconvert2/Temperature Conversion  IU=K  OU=C
  Bus Element Out3 : Outport  PortName=dpressure  Element=timestamp
  Bus Element Out4 : Outport  PortName=dpressure  Element=timestamp_sample
  Bus Element Out5 : Outport  PortName=dpressure  Element=device_id
  Bus Element Out : Outport  PortName=dpressure  Element=differential_pressure_pa
  Bus Element Out6 : Outport  PortName=dpressure  Element=temperature
  Bus Element Out1 : Outport  PortName=dpressure  Element=error_count
  wires:
  Data Type Conversion1/1 -> Bus Element Out/1
  Bus Element In1/1 -> Data Type Conversion1/1
  Data Type Conversion/1 -> Temperature Conversion/1
  Temperature Conversion/1 -> Bus Element Out6/1
  Bus Element In2/1 -> Data Type Conversion/1
  Constant/1 -> Bus Element Out5/1
  Gain/1 -> Signal Specification3/1
  Signal Specification3/1 -> Bus Element Out3/1, Bus Element Out4/1
  Clock/1 -> Gain/1
  Constant1/1 -> Bus Element Out1/1

== system vtol50kg_airframe/sensor/baro ==
  Bus Element In2 : Inport  PortName=state  Element=environ.atmosphere.temperature
  Bus Element In1 : Inport  PortName=state  Element=environ.atmosphere.pressure
  Clock : Clock
  Constant : Constant  Value=0  OutDataTypeStr=uint32
  Constant1 : Constant  Value=0  OutDataTypeStr=uint32
  Data Type Conversion : DataTypeConversion  OutDataTypeStr=single  SaturateOnIntegerOverflow=off  RndMeth=Floor
  Data Type Conversion1 : DataTypeConversion  OutDataTypeStr=single  SaturateOnIntegerOverflow=off  RndMeth=Floor
  Gain : Gain  Gain=1e6  OutDataTypeStr=uint64
  Signal Specification3 : SignalSpecification  Unit=µs
  Temperature Conversion : aerolibconvert2/Temperature Conversion  IU=K  OU=C
  Bus Element Out3 : Outport  PortName=baro  Element=timestamp
  Bus Element Out4 : Outport  PortName=baro  Element=timestamp_sample
  Bus Element Out5 : Outport  PortName=baro  Element=device_id
  Bus Element Out : Outport  PortName=baro  Element=pressure
  Bus Element Out6 : Outport  PortName=baro  Element=temperature
  Bus Element Out7 : Outport  PortName=baro  Element=error_count
  wires:
  Clock/1 -> Gain/1
  Signal Specification3/1 -> Bus Element Out4/1, Bus Element Out3/1
  Gain/1 -> Signal Specification3/1
  Constant/1 -> Bus Element Out5/1
  Constant1/1 -> Bus Element Out7/1
  Bus Element In2/1 -> Data Type Conversion/1
  Temperature Conversion/1 -> Bus Element Out6/1
  Data Type Conversion/1 -> Temperature Conversion/1
  Bus Element In1/1 -> Data Type Conversion1/1
  Data Type Conversion1/1 -> Bus Element Out/1

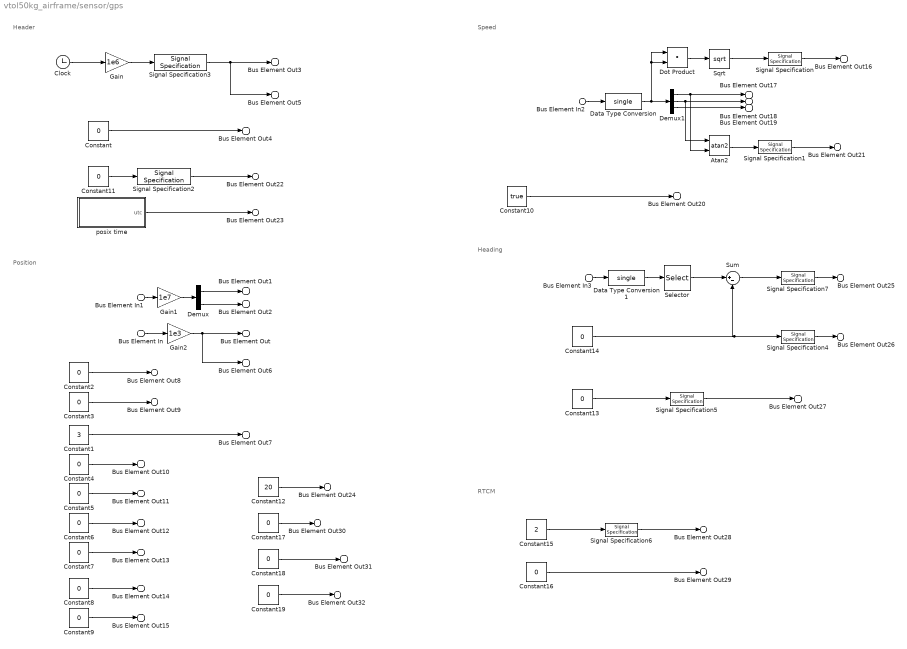
== system vtol50kg_airframe/sensor/gps ==
  note: RTCM
  note: Heading
  note: Speed
  note: Header
  note: Position
  Bus Element In : Inport  PortName=state  Element=aircraft.position.alt
  Bus Element In1 : Inport  PortName=state  Element=aircraft.position.lat_lon
  Bus Element In2 : Inport  PortName=state  Element=aircraft.position.vn_ve_vd
  Bus Element In3 : Inport  PortName=state  Element=aircraft.attitude.phi_theta_psi
  Atan2 : Trigonometry  Operator=atan2
  Clock : Clock
  Constant : Constant  Value=0  OutDataTypeStr=uint32
  Constant1 : Constant  Value=3  OutDataTypeStr=uint8
  Constant10 : Constant  Value=true  OutDataTypeStr=boolean
  Constant11 : Constant  Value=0  OutDataTypeStr=uint32
  Constant12 : Constant  Value=20  OutDataTypeStr=uint8
  Constant{2..7,13..14} (8 alike) : Constant  Value=0  OutDataTypeStr=single
  Constant15 : Constant  Value=2  OutDataTypeStr=single
  Constant16 : Constant  Value=0  OutDataTypeStr=uint8
  Constant17 : Constant  Value=0  OutDataTypeStr=uint8
  Constant18 : Constant  Value=0  OutDataTypeStr=int32
  Constant19 : Constant  Value=0  OutDataTypeStr=uint8
  Constant8 : Constant  Value=0  OutDataTypeStr=int32
  Constant9 : Constant  Value=0  OutDataTypeStr=uint16
  Data Type Conversion : DataTypeConversion  OutDataTypeStr=single  SaturateOnIntegerOverflow=off  RndMeth=Floor
  Data Type Conversion1 : DataTypeConversion  OutDataTypeStr=single  SaturateOnIntegerOverflow=off  RndMeth=Floor
  Demux : Demux  Outputs=2
  Demux1 : Demux  Outputs=3
  Dot Product : DotProduct  OutDataTypeStr=Inherit: Inherit via internal rule
  Gain : Gain  Gain=1e6  OutDataTypeStr=uint64
  Gain1 : Gain  Gain=1e7  OutDataTypeStr=int32
  Gain2 : Gain  Gain=1e3  OutDataTypeStr=int32
  Selector : Selector  InputPortWidth=3  IndexOptions=Index vector (dialog)  Indices=3  OutputSizes=1
  Signal Specification : SignalSpecification  Unit=m/s
  Signal Specification{1,4..5,7} (4 alike) : SignalSpecification  Unit=rad
  Signal Specification2 : SignalSpecification  Unit=ms
  Signal Specification3 : SignalSpecification  Unit=µs
  Signal Specification6 : SignalSpecification  Unit=Hz
  Sqrt : Sqrt
  Sum : Sum  Inputs=|+-
  posix time : Subsystem
  Bus Element Out3 : Outport  PortName=gps  Element=timestamp
  Bus Element Out5 : Outport  PortName=gps  Element=timestamp_sample
  Bus Element Out4 : Outport  PortName=gps  Element=device_id
  Bus Element Out1 : Outport  PortName=gps  Element=lat
  Bus Element Out2 : Outport  PortName=gps  Element=lon
  Bus Element Out : Outport  PortName=gps  Element=alt
  Bus Element Out6 : Outport  PortName=gps  Element=alt_ellipsoid
  Bus Element Out8 : Outport  PortName=gps  Element=s_variance_m_s
  Bus Element Out9 : Outport  PortName=gps  Element=c_variance_rad
  Bus Element Out7 : Outport  PortName=gps  Element=fix_type
  Bus Element Out10 : Outport  PortName=gps  Element=eph
  Bus Element Out11 : Outport  PortName=gps  Element=epv
  Bus Element Out12 : Outport  PortName=gps  Element=hdop
  Bus Element Out13 : Outport  PortName=gps  Element=vdop
  Bus Element Out14 : Outport  PortName=gps  Element=noise_per_ms
  Bus Element Out15 : Outport  PortName=gps  Element=automatic_gain_control
  Bus Element Out30 : Outport  PortName=gps  Element=jamming_state
  Bus Element Out31 : Outport  PortName=gps  Element=jamming_indicator
  Bus Element Out32 : Outport  PortName=gps  Element=spoofing_state
  Bus Element Out16 : Outport  PortName=gps  Element=vel_m_s
  Bus Element Out17 : Outport  PortName=gps  Element=vel_n_m_s
  Bus Element Out18 : Outport  PortName=gps  Element=vel_e_m_s
  Bus Element Out19 : Outport  PortName=gps  Element=vel_d_m_s
  Bus Element Out21 : Outport  PortName=gps  Element=cog_rad
  Bus Element Out20 : Outport  PortName=gps  Element=vel_ned_valid
  Bus Element Out22 : Outport  PortName=gps  Element=timestamp_time_relative
  Bus Element Out23 : Outport  PortName=gps  Element=time_utc_usec
  Bus Element Out24 : Outport  PortName=gps  Element=satellites_used
  Bus Element Out25 : Outport  PortName=gps  Element=heading
  Bus Element Out26 : Outport  PortName=gps  Element=heading_offset
  Bus Element Out27 : Outport  PortName=gps  Element=heading_accuracy
  Bus Element Out28 : Outport  PortName=gps  Element=rtcm_injection_rate
  Bus Element Out29 : Outport  PortName=gps  Element=selected_rtcm_instance
  wires:
  Bus Element In/1 -> Gain2/1
  Bus Element In1/1 -> Gain1/1
  Demux/1 -> Bus Element Out1/1
  Demux/2 -> Bus Element Out2/1
  Clock/1 -> Gain/1
  Gain/1 -> Signal Specification3/1
  Constant/1 -> Bus Element Out4/1
  Gain1/1 -> Demux/1
  Gain2/1 -> Bus Element Out6/1, Bus Element Out/1
  Constant1/1 -> Bus Element Out7/1
  Constant2/1 -> Bus Element Out8/1
  Constant3/1 -> Bus Element Out9/1
  Constant4/1 -> Bus Element Out10/1
  Constant5/1 -> Bus Element Out11/1
  Constant7/1 -> Bus Element Out13/1
  Constant6/1 -> Bus Element Out12/1
  Constant9/1 -> Bus Element Out15/1
  Constant8/1 -> Bus Element Out14/1
  Bus Element In2/1 -> Data Type Conversion/1
  Demux1/1 -> Atan2/2, Bus Element Out17/1
  Demux1/2 -> Atan2/1, Bus Element Out18/1
  Demux1/3 -> Bus Element Out19/1
  Constant10/1 -> Bus Element Out20/1
  Atan2/1 -> Signal Specification1/1
  Sqrt/1 -> Signal Specification/1
  Dot Product/1 -> Sqrt/1
  Data Type Conversion/1 -> Demux1/1, Dot Product/1, Dot Product/2
  Signal Specification/1 -> Bus Element Out16/1
  Signal Specification1/1 -> Bus Element Out21/1
  Constant12/1 -> Bus Element Out24/1
  Bus Element In3/1 -> Data Type Conversion1/1
  Constant14/1 -> Sum/2, Signal Specification4/1
  Selector/1 -> Sum/1
  Constant13/1 -> Signal Specification5/1
  Sum/1 -> Signal Specification7/1
  Constant15/1 -> Signal Specification6/1
  Constant16/1 -> Bus Element Out29/1
  Constant11/1 -> Signal Specification2/1
  posix time/1(utc) -> Bus Element Out23/1
  Signal Specification2/1 -> Bus Element Out22/1
  Signal Specification3/1 -> Bus Element Out5/1, Bus Element Out3/1
  Signal Specification4/1 -> Bus Element Out26/1
  Signal Specification5/1 -> Bus Element Out27/1
  Signal Specification6/1 -> Bus Element Out28/1
  Constant17/1 -> Bus Element Out30/1
  Constant18/1 -> Bus Element Out31/1
  Constant19/1 -> Bus Element Out32/1
  Signal Specification7/1 -> Bus Element Out25/1
  Data Type Conversion1/1 -> Selector/1

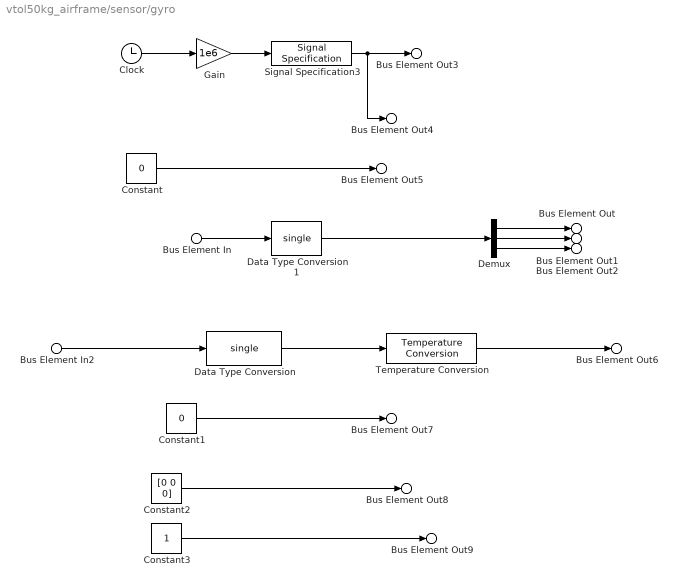
== system vtol50kg_airframe/sensor/gyro ==
  Bus Element In2 : Inport  PortName=state  Element=environ.atmosphere.temperature
  Bus Element In : Inport  PortName=state  Element=aircraft.attitude.p_q_r
  Clock : Clock
  Constant : Constant  Value=0  OutDataTypeStr=uint32
  Constant1 : Constant  Value=0  OutDataTypeStr=uint32
  Constant2 : Constant  Value=[0 0 0]  OutDataTypeStr=uint8
  Constant3 : Constant  OutDataTypeStr=uint8
  Data Type Conversion : DataTypeConversion  OutDataTypeStr=single  SaturateOnIntegerOverflow=off  RndMeth=Floor
  Data Type Conversion1 : DataTypeConversion  OutDataTypeStr=single  SaturateOnIntegerOverflow=off  RndMeth=Floor
  Demux : Demux  Outputs=3
  Gain : Gain  Gain=1e6  OutDataTypeStr=uint64
  Signal Specification3 : SignalSpecification  Unit=µs
  Temperature Conversion : aerolibconvert2/Temperature Conversion  IU=K  OU=C
  Bus Element Out3 : Outport  PortName=gyro  Element=timestamp
  Bus Element Out4 : Outport  PortName=gyro  Element=timestamp_sample
  Bus Element Out5 : Outport  PortName=gyro  Element=device_id
  Bus Element Out : Outport  PortName=gyro  Element=x
  Bus Element Out1 : Outport  PortName=gyro  Element=y
  Bus Element Out2 : Outport  PortName=gyro  Element=z
  Bus Element Out6 : Outport  PortName=gyro  Element=temperature
  Bus Element Out7 : Outport  PortName=gyro  Element=error_count
  Bus Element Out8 : Outport  PortName=gyro  Element=clip_counter
  Bus Element Out9 : Outport  PortName=gyro  Element=samples
  wires:
  Data Type Conversion1/1 -> Demux/1
  Data Type Conversion/1 -> Temperature Conversion/1
  Temperature Conversion/1 -> Bus Element Out6/1
  Bus Element In2/1 -> Data Type Conversion/1
  Constant1/1 -> Bus Element Out7/1
  Constant/1 -> Bus Element Out5/1
  Gain/1 -> Signal Specification3/1
  Signal Specification3/1 -> Bus Element Out3/1, Bus Element Out4/1
  Clock/1 -> Gain/1
  Demux/3 -> Bus Element Out2/1
  Demux/2 -> Bus Element Out1/1
  Demux/1 -> Bus Element Out/1
  Bus Element In/1 -> Data Type Conversion1/1
  Constant2/1 -> Bus Element Out8/1
  Constant3/1 -> Bus Element Out9/1

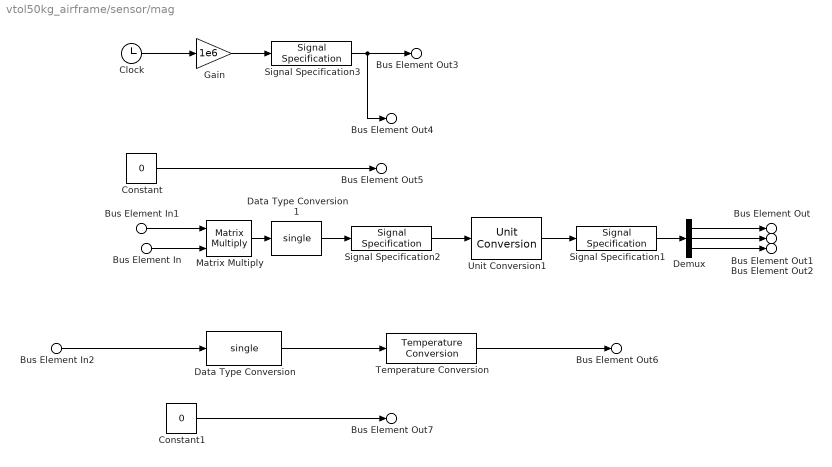
== system vtol50kg_airframe/sensor/mag ==
  Bus Element In : Inport  PortName=state  Element=environ.magnetic.xyz
  Bus Element In2 : Inport  PortName=state  Element=environ.atmosphere.temperature
  Bus Element In1 : Inport  PortName=state  Element=aircraft.attitude.Rbe
  Clock : Clock
  Constant : Constant  Value=0  OutDataTypeStr=uint32
  Constant1 : Constant  Value=0  OutDataTypeStr=uint32
  Data Type Conversion : DataTypeConversion  OutDataTypeStr=single  SaturateOnIntegerOverflow=off  RndMeth=Floor
  Data Type Conversion1 : DataTypeConversion  OutDataTypeStr=single  SaturateOnIntegerOverflow=off  RndMeth=Floor
  Demux : Demux  Outputs=3
  Gain : Gain  Gain=1e6  OutDataTypeStr=uint64
  Matrix Multiply : Product  Multiplication=Matrix(*)
  Signal Specification1 : SignalSpecification  Unit=G
  Signal Specification2 : SignalSpecification  Unit=nT
  Signal Specification3 : SignalSpecification  Unit=µs
  Temperature Conversion : aerolibconvert2/Temperature Conversion  IU=K  OU=C
  Unit Conversion1 : UnitConversion
  Bus Element Out3 : Outport  PortName=mag  Element=timestamp
  Bus Element Out4 : Outport  PortName=mag  Element=timestamp_sample
  Bus Element Out5 : Outport  PortName=mag  Element=device_id
  Bus Element Out : Outport  PortName=mag  Element=x
  Bus Element Out1 : Outport  PortName=mag  Element=y
  Bus Element Out2 : Outport  PortName=mag  Element=z
  Bus Element Out6 : Outport  PortName=mag  Element=temperature
  Bus Element Out7 : Outport  PortName=mag  Element=error_count
  wires:
  Bus Element In/1 -> Matrix Multiply/2
  Bus Element In1/1 -> Matrix Multiply/1
  Matrix Multiply/1 -> Data Type Conversion1/1
  Demux/1 -> Bus Element Out/1
  Demux/2 -> Bus Element Out1/1
  Demux/3 -> Bus Element Out2/1
  Clock/1 -> Gain/1
  Signal Specification3/1 -> Bus Element Out4/1, Bus Element Out3/1
  Gain/1 -> Signal Specification3/1
  Constant/1 -> Bus Element Out5/1
  Constant1/1 -> Bus Element Out7/1
  Bus Element In2/1 -> Data Type Conversion/1
  Temperature Conversion/1 -> Bus Element Out6/1
  Data Type Conversion/1 -> Temperature Conversion/1
  Data Type Conversion1/1 -> Signal Specification2/1
  Signal Specification1/1 -> Demux/1
  Unit Conversion1/1 -> Signal Specification1/1
  Signal Specification2/1 -> Unit Conversion1/1

== system vtol50kg_airframe/state/Variant Subsystem ==
  note: 1) Add Subsystem or Model blocks as valid variant choices.
      | 2) You cannot connect blocks at this level. At simulation, connectivity is automatically
      | determined, based on the active variant and port name matching.
  h(m) : Inport
  μ(deg) : Inport  Port=2
  l(deg) : Inport  Port=3
  None : Subsystem  VariantControl=true
  WMM2020 : Subsystem  VariantControl=false
  XYZ(nT) : Outport
  H(nT) : Outport  Port=2
  D(deg) : Outport  Port=3
  I(deg) : Outport  Port=4
  F(nT) : Outport  Port=5

== system vtol50kg_airframe/actuator/engine/Subsystem ==
  rho : Inport
  throttle : Inport  Port=2
  1-D Lookup Table2 : Lookup_n-D  NumberOfTableDimensions=1  BreakpointsForDimension1=engine.torque.delta  IndexSearchMethod=Linear search  BeginIndexSearchUsingPreviousIndexResult=on  Table=engine.torque.power  ExtrapMethod=Clip  InternalRulePriority=Speed  RndMeth=Simplest
  Power_alt : MATLAB Function  TreatAsAtomicUnit=on
  power : Outport
  wires:
  throttle/1 -> 1-D Lookup Table2/1
  rho/1 -> Power_alt/1(rho)
  1-D Lookup Table2/1 -> Power_alt/2(power)
  Power_alt/1(power_h) -> power/1

== system vtol50kg_airframe/actuator/engine/Subsystem1 ==
  power : Inport
  va : Inport  Port=2
  alt : Inport  Port=3
  rho : Inport  Port=4
  throttle : Inport  Port=5
  rpm : Inport  Port=6
  1-D Lookup Table1 : Lookup_n-D  NumberOfTableDimensions=1  BreakpointsForDimension1=engine.thrust.delta  IndexSearchMethod=Linear search  BeginIndexSearchUsingPreviousIndexResult=on  Table=engine.thrust.force  ExtrapMethod=Clip  InternalRulePriority=Speed  RndMeth=Simplest
  Constant2 : Constant  Value=engine.propeller_dia
  Dynamic_thrust : MATLAB Function  TreatAsAtomicUnit=on
  dynamic_thrust : Outport
  wires:
  power/1 -> Dynamic_thrust/2(power)
  1-D Lookup Table1/1 -> Dynamic_thrust/3(thrust)  "thrust"
  rpm/1 -> Dynamic_thrust/1(rpm)
  va/1 -> Dynamic_thrust/5(va)
  Constant2/1 -> Dynamic_thrust/7(blade_D)
  throttle/1 -> 1-D Lookup Table1/1
  rho/1 -> Dynamic_thrust/6(rho)
  Dynamic_thrust/1(thrust_d) -> dynamic_thrust/1
  alt/1 -> Dynamic_thrust/4(alt)
